simulink model "dobleterminado"  (R2022b)
settings: Solver=VariableStepAuto  StartTime=0.0  StopTime=10.0  MaxStep=0.00001  RelTol=1e-3
undefined symbols (not defined in the file): g, l1, l2, m1, m2
settings Model: Creator=mluser  LastModifiedBy=mluser

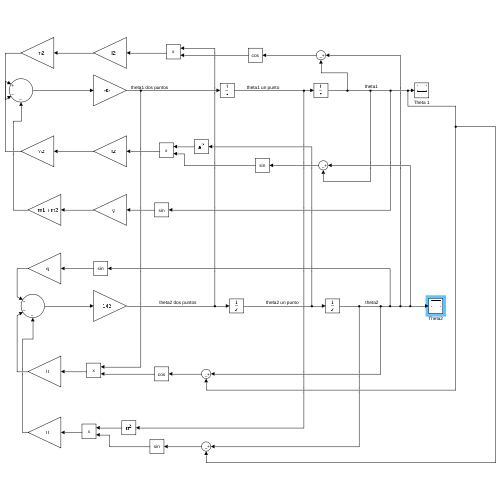
[thumbnail: Simulink's stored preview of the top-level diagram]
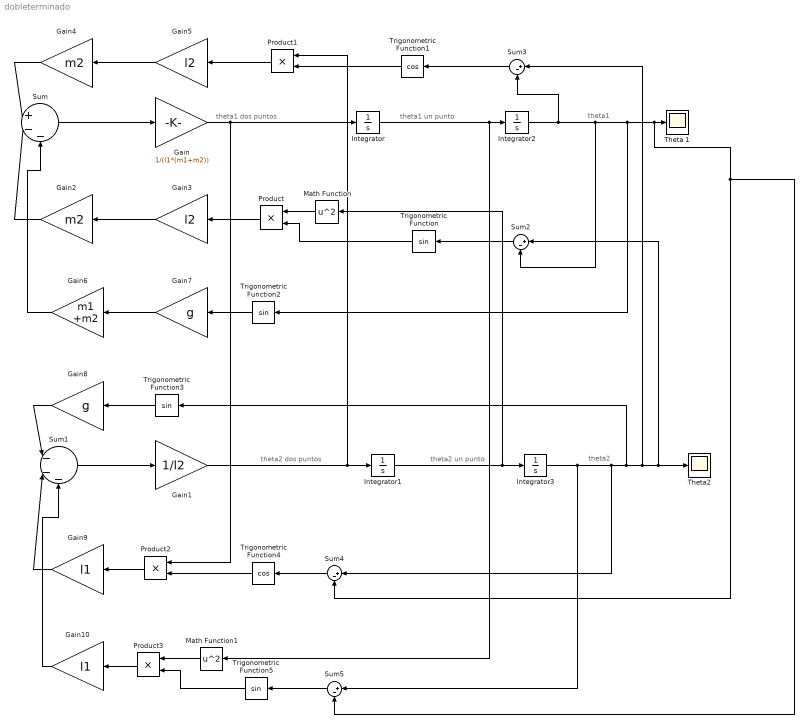
== system dobleterminado ==
  note: theta1
  note: theta1 un punto
  note: theta1 dos puntos
  note: theta2 dos puntos
  note: theta2 un punto
  note: theta2
  Gain : Gain  Gain=1/(l1*(m1+m2))
  Gain1 : Gain  Gain=1/l2
  Gain10 : Gain  Gain=l1
  Gain2 : Gain  Gain=m2
  Gain3 : Gain  Gain=l2
  Gain4 : Gain  Gain=m2
  Gain5 : Gain  Gain=l2
  Gain6 : Gain  Gain=m1 +m2
  Gain7 : Gain  Gain=g
  Gain8 : Gain  Gain=g
  Gain9 : Gain  Gain=l1
  Integrator : Integrator
  Integrator1 : Integrator
  Integrator2 : Integrator
  Integrator3 : Integrator  InitialCondition=35*(pi/180)
  Math Function : Math  Operator=square
  Math Function1 : Math  Operator=square
  Product{,1..3} (4 alike) : Product
  Sum : Sum  Inputs=|+--
  Sum1 : Sum  Inputs=|---
  Sum{2..5} (4 alike) : Sum  Inputs=|+-
  Theta 1 : Scope
  Theta2 : Scope
  Trigonometric Function{,2..3,5} (4 alike) : Trigonometry
  Trigonometric Function1 : Trigonometry  Operator=cos
  Trigonometric Function4 : Trigonometry  Operator=cos
  wires:
  Gain/1 -> Integrator/1, Product2/1
  Gain1/1 -> Integrator1/1, Product1/1
  Integrator/1 -> Math Function1/1, Integrator2/1
  Integrator1/1 -> Math Function/1, Integrator3/1
  Integrator3/1 -> Sum5/1, Sum4/1, Trigonometric Function3/1, Sum3/1, Sum2/1, Theta2/1
  Sum1/1 -> Gain1/1
  Sum/1 -> Gain/1
  Gain2/1 -> Sum/1
  Gain3/1 -> Gain2/1
  Product/1 -> Gain3/1
  Math Function/1 -> Product/1
  Trigonometric Function/1 -> Product/2
  Sum2/1 -> Trigonometric Function/1
  Gain4/1 -> Sum/2
  Gain5/1 -> Gain4/1
  Product1/1 -> Gain5/1
  Sum3/1 -> Trigonometric Function1/1
  Gain6/1 -> Sum/3
  Gain7/1 -> Gain6/1
  Trigonometric Function2/1 -> Gain7/1
  Gain8/1 -> Sum1/1
  Trigonometric Function3/1 -> Gain8/1
  Gain9/1 -> Sum1/2
  Product2/1 -> Gain9/1
  Trigonometric Function1/1 -> Product1/2
  Trigonometric Function4/1 -> Product2/2
  Sum4/1 -> Trigonometric Function4/1
  Gain10/1 -> Sum1/3
  Product3/1 -> Gain10/1
  Math Function1/1 -> Product3/1
  Trigonometric Function5/1 -> Product3/2
  Sum5/1 -> Trigonometric Function5/1
  Integrator2/1 -> Trigonometric Function2/1, Sum5/2, Sum4/2, Theta 1/1, Sum2/2, Sum3/2
